simulink model "pumpa"  (R2017b)
settings: Solver=VariableStepAuto  StartTime=0.0  StopTime=5500.0  RelTol=1e-3
libraries: simulink x1
settings Model: Creator=DT User  LastModifiedBy=DT User

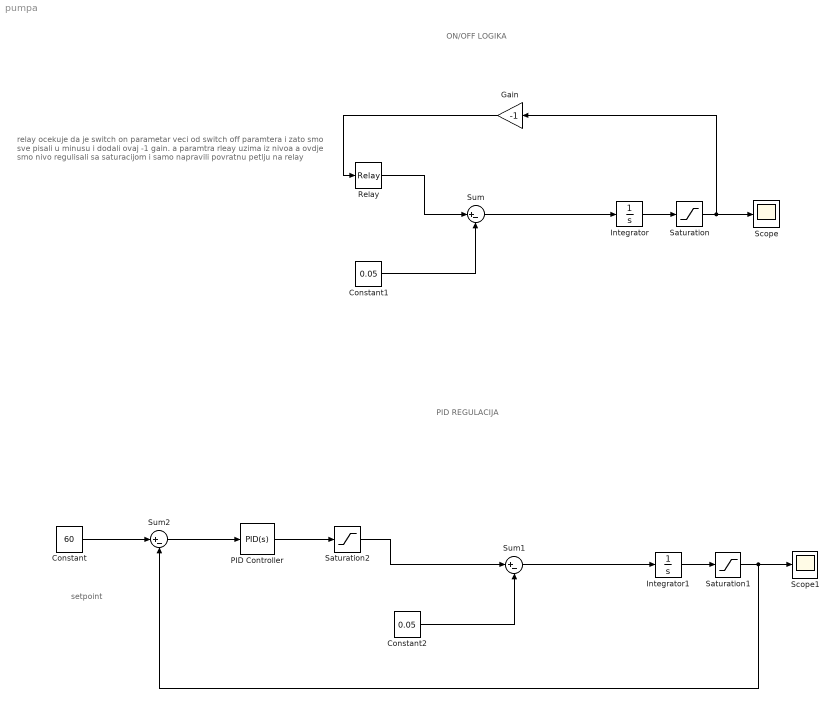
== system pumpa ==
  note: setpoint
  note: PID REGULACIJA
  note: ON/OFF LOGIKA
  note: relay ocekuje da je switch on parametar veci od switch off paramtera i
      | zato smo sve pisali u minusu i dodali ovaj -1 gain.
      | a paramtra rleay uzima iz nivoa
      | a ovdje smo nivo regulisali sa
      | saturacijom i samo napravili
      | povratnu petlju na relay
  Constant : Constant  Value=60
  Constant1 : Constant  Value=0.05
  Constant2 : Constant  Value=0.05
  Gain : Gain  Gain=-1
  Integrator : Integrator  InitialCondition=50
  Integrator1 : Integrator  InitialCondition=50
  PID Controller : simulink/Continuous/PID Controller  Controller=PID  TimeDomain=Continuous-time  SampleTime=-1  IntegratorMethod=Forward Euler  FilterMethod=Forward Euler  Form=Parallel  UseFilter=on  ControllerParametersSource=internal  P=0.01  I=0.0001  D=0  N=100  InitialConditionSource=internal  InitialConditionForIntegrator=0  InitialConditionForFilter=0  ExternalReset=none  LimitOutput=off  UpperSaturationLimit=inf  LowerSaturationLimit=-inf  LinearizeAsGain=on  AntiWindupMode=none  Kb=1  TrackingMode=off  Kt=1  PParamMin=[]  PParamMax=[]  IParamMin=[]  IParamMax=[]  DParamMin=[]  DParamMax=[]  NParamMin=[]  NParamMax=[]  KbParamMin=[]  KbParamMax=[]  KtParamMin=[]  KtParamMax=[]  POutMin=[]  POutMax=[]  IOutMin=[]  IOutMax=[]  DOutMin=[]  DOutMax=[]  NOutMin=[]  NOutMax=[]  KbOutMin=[]  KbOutMax=[]  KtOutMin=[]  KtOutMax=[]  IntegratorOutMin=[]  IntegratorOutMax=[]  FilterOutMin=[]  FilterOutMax=[]  SumOutMin=[]  SumOutMax=[]  SumI1OutMin=[]  SumI1OutMax=[]  SumI2OutMin=[]  SumI2OutMax=[]  SumI3OutMin=[]  SumI3OutMax=[]  SumDOutMin=[]  SumDOutMax=[]  SaturationOutMin=[]  SaturationOutMax=[]  IntegratorContinuousStateAttributes=''  IntegratorStateMustResolveToSignalObject=off  IntegratorRTWStateStorageClass=Auto  FilterContinuousStateAttributes=''  FilterStateMustResolveToSignalObject=off  FilterRTWStateStorageClass=Auto  DifferentiatorICPrevScaledInput=0  DifferentiatorOutMin=[]  DifferentiatorOutMax=[]  InitialConditionSetting=State (most efficient)  FilterDiffOutCoefMin=[]  FilterDiffOutCoefMax=[]  SumDenOutMin=[]  SumDenOutMax=[]  SumNumOutMin=[]  SumNumOutMax=[]  ReciprocalOutMin=[]  ReciprocalOutMax=[]  DivideOutMin=[]  DivideOutMax=[]  TunerSelectOption=Transfer Function Based (PID Tuner App)
  Relay : Relay  OnSwitchValue=-30  OffSwitchValue=-80  OnOutputValue=0.08
  Saturation : Saturate  UpperLimit=100  LowerLimit=0
  Saturation1 : Saturate  UpperLimit=100  LowerLimit=0
  Saturation2 : Saturate  UpperLimit=0.08  LowerLimit=0
  Scope : Scope
  Scope1 : Scope
  Sum : Sum  Inputs=|+-
  Sum1 : Sum  Inputs=|+-
  Sum2 : Sum  Inputs=|+-
  wires:
  Sum/1 -> Integrator/1
  Integrator/1 -> Saturation/1
  Relay/1 -> Sum/1
  Constant1/1 -> Sum/2
  Saturation/1 -> Gain/1, Scope/1
  Gain/1 -> Relay/1
  Sum1/1 -> Integrator1/1
  Constant2/1 -> Sum1/2
  Integrator1/1 -> Saturation1/1
  Saturation1/1 -> Sum2/2, Scope1/1
  Constant/1 -> Sum2/1
  Sum2/1 -> PID Controller/1
  PID Controller/1 -> Saturation2/1
  Saturation2/1 -> Sum1/1
